simulink model "KVHTestMath01"  (Simulink 7.9)
settings: Solver=FixedStepDiscrete  StartTime=0.0  StopTime=T(end)  FixedStep=0.001  RelTol=1e-3
InitFcn:
  | T = (0:length(DeltaAngle)-1)'*0.001;
  | TDeltaAngle = [T DeltaAngle];
  | TAcceleration = [T Acceleration];
  | TStatus = [T Status];
  | TValid = [T Valid];
StopFcn:
  | ZYX = yout(:,1:3);
  | R=yout(:,4:12);
  | 
  | figure(1);
  | plot(T,ZYX*180/pi); hold on;
  | plot(T,Status, 'm'); hold off;
libraries: simulink x2
settings Model: Creator=bgbuss  LastModifiedBy=bgbuss
settings DataIOCC: LimitDataPoints=off

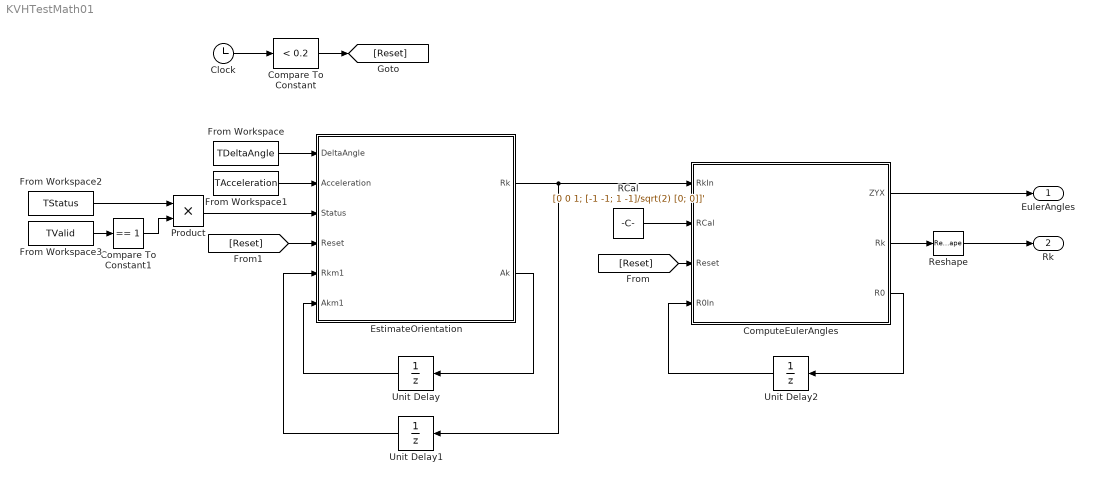
== system KVHTestMath01 ==
  Clock : Clock
  Compare To Constant : simulink/Logic and Bit Operations/Compare To Constant  relop=<  const=0.2  OutDataTypeStr=uint8
  Compare To Constant1 : simulink/Logic and Bit Operations/Compare To Constant  relop===  const=1  OutDataTypeStr=uint8
  ComputeEulerAngles : MATLAB Function  TreatAsAtomicUnit=on
  EstimateOrientation : MATLAB Function  TreatAsAtomicUnit=on
  From Workspace : FromWorkspace  VariableName=TDeltaAngle  SampleTime=0  Interpolate=off  OutputAfterFinalValue=Holding final value
  From Workspace1 : FromWorkspace  VariableName=TAcceleration  SampleTime=0  Interpolate=off  OutputAfterFinalValue=Holding final value
  From Workspace2 : FromWorkspace  VariableName=TStatus  SampleTime=0  Interpolate=off  OutputAfterFinalValue=Holding final value
  From Workspace3 : FromWorkspace  VariableName=TValid  SampleTime=0  Interpolate=off  OutputAfterFinalValue=Holding final value
  Product : Product  RndMeth=Zero
  RCal : Constant  Value=[0 0 1; [-1 -1; 1 -1]/sqrt(2) [0; 0]]'
  Reshape : Reshape
  Unit Delay : UnitDelay  X0=[0; 0; 0]  SampleTime=-1
  Unit Delay1 : UnitDelay  X0=zeros(3,3)  SampleTime=-1
  Unit Delay2 : UnitDelay  X0=zeros(3,3)  SampleTime=-1
  EulerAngles : Outport
  Rk : Outport  Port=2
  wires:
  EstimateOrientation/2(Ak) -> Unit Delay/1
  Unit Delay/1 -> EstimateOrientation/6(Akm1)
  EstimateOrientation/1(Rk) -> Unit Delay1/1, ComputeEulerAngles/1(RkIn)
  Unit Delay1/1 -> EstimateOrientation/5(Rkm1)
  [Reset] -> EstimateOrientation/4(Reset)
  RCal/1 -> ComputeEulerAngles/2(RCal)
  Unit Delay2/1 -> ComputeEulerAngles/4(R0In)
  ComputeEulerAngles/1(ZYX) -> EulerAngles/1
  ComputeEulerAngles/3(R0) -> Unit Delay2/1
  ComputeEulerAngles/2(Rk) -> Reshape/1
  [Reset] -> ComputeEulerAngles/3(Reset)
  From Workspace/1 -> EstimateOrientation/1(DeltaAngle)
  From Workspace1/1 -> EstimateOrientation/2(Acceleration)
  Clock/1 -> Compare To Constant/1
  Compare To Constant/1 -> [Reset]
  From Workspace2/1 -> Product/1
  Reshape/1 -> Rk/1
  Product/1 -> EstimateOrientation/3(Status)
  From Workspace3/1 -> Compare To Constant1/1
  Compare To Constant1/1 -> Product/2

== matlab function ComputeEulerAngles ==
  data: RkIn input double; RCal input double; Reset input double; R0In input double; ZYX output double; Rk output double; R0 output double
function [ZYX, Rk, R0] = fcn(RkIn, RCal, Reset, R0In) %#codegen
    % Convert from IMU frame to robot frame and compute Euler angles. The
    % yaw angle is zeroed whenever (Reset) is true.
        
    if (Reset)
        % Compute the rotation matrix which zeros the initial yaw
        qT0 = M_to_ZYX(RkIn*RCal);
        R0  = Rz(-qT0(1));
    else
        R0 = R0In;
    end
    
    % Transform from IMU to robot frame and zero initial yaw
    Rk = R0*RkIn*RCal;
    
    % Convert Rk to ZYX Euler angles
    ZYX = M_to_ZYX(Rk);
end

function R = Rz(t)
    R = [cos(t) -sin(t) 0; sin(t) cos(t) 0; 0 0 1];
end

== matlab function EstimateOrientation ==
  data: DeltaAngle input double; Acceleration input double; Status input double; Reset input double; Rk output double; Rkm1 input double; Akm1 input double; Ak output double
function [Rk, Ak] = fcn(DeltaAngle,Acceleration,Status,Reset,Rkm1,Akm1) %#codegen
    [Rk, Ak] = estimateOrientation(DeltaAngle,Acceleration,Rkm1,Akm1,Status,Reset);
end
